simulink model "robot2018b"  (R2018b)
settings: Solver=VariableStepAuto  StartTime=0.0  StopTime=10  RelTol=1e-3
libraries: robotmobilelib x1, simulink x1
settings Model: Creator=kika  LastModifiedBy=kika
settings DataIOCC: ReturnWorkspaceOutputs=on

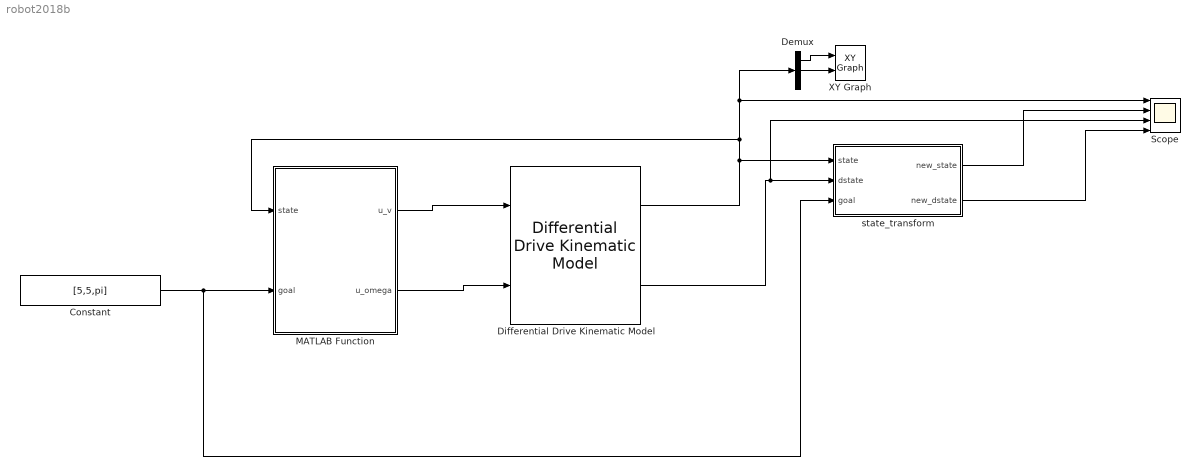
== system robot2018b ==
  Constant : Constant  Value=[5,5,pi]
  Demux : Demux  Outputs=3
  Differential Drive Kinematic Model : robotmobilelib/Differential Drive Kinematic Model  VehicleInputs=Vehicle Speed & Heading Angular Velocity  WheelRadius=0.05  WheelSpeedRange=[-inf inf]  TrackWidth=0.2  InitialState=[0, 0, 0]'  SimulateUsing=Interpreted execution
      settings: SourceProductName=Robotics System Toolbox
  MATLAB Function : MATLAB Function  TreatAsAtomicUnit=on
  Scope : Scope  NumInputPorts=4
  XY Graph : simulink/Sinks/XY Graph  xmin=-10  xmax=10  ymin=-10  ymax=10  st=-1
  state_transform : MATLAB Function  TreatAsAtomicUnit=on
  wires:
  Differential Drive Kinematic Model/1 -> MATLAB Function/1(state), Demux/1, Scope/1, state_transform/1(state)
  Demux/1 -> XY Graph/1
  Demux/2 -> XY Graph/2
  MATLAB Function/1(u_v) -> Differential Drive Kinematic Model/1
  MATLAB Function/2(u_omega) -> Differential Drive Kinematic Model/2
  Constant/1 -> state_transform/3(goal), MATLAB Function/2(goal)
  Differential Drive Kinematic Model/2 -> Scope/3, state_transform/2(dstate)
  state_transform/1(new_state) -> Scope/2
  state_transform/2(new_dstate) -> Scope/4

== matlab function robot2018b/state_transform ==
  data: state input; new_state output; dstate input; new_dstate output; goal input
function [new_state, new_dstate]= fcn(state, dstate, goal)
    
    x_goal = goal(1);
    y_goal = goal(2);
    theta_goal = goal(3);


    % initial transfrom
    R = [
        cos(theta_goal), -sin(theta_goal), 0;
        sin(theta_goal),cos(theta_goal), 0;
        0,0,1
    ];
    
    p = [x_goal, y_goal, 0]';
    
    
    T = [
        R, p;
        0,0,0,1
    ];
    
    
    new_state = inv(T) * [state(1), state(2), 0, 1]';

    
    iT = inv(T);
    R = iT(1:3, 1:3);
    p = iT(1:3, 4);

    Ad = [
        R,            zeros(size(R));
       zeros(size(R)),     R
    ];

    new_dstate = Ad' * [dstate(1), dstate(2), 0, 0, 0, dstate(3)]';%  skew(p) * R

== matlab function robot2018b/MATLAB Function ==
  data: state input; u_v output; u_omega output; goal input
function [u_v, u_omega] = controller(state, goal)

    x = state(1);
    y = state(2);
    theta = state(3);
    
    x_goal = goal(1);
    y_goal = goal(2);
%     theta_goal = goal(3);
    
    e_x = x_goal - x;
    e_y = y_goal - y;
    
    dist_to_goal = sqrt(e_x^2 + e_y^2);
    
    e_theta = -atan2(e_y, e_x) + theta;
    if theta > pi
        e_theta = -atan2(e_y, e_x) + theta - 2 * pi;
    end
        

    k = 1;
    k_a = 5;

    % go to 
    u_v = k * dist_to_goal * cos(e_theta);
    u_omega = - k_a * e_theta;
